simulink model "Part E"  (R2022b)
settings: Solver=VariableStepAuto  StartTime=0.0  StopTime=10.0  RelTol=1e-3
libraries: commanapbnd3 x4
settings Model: Creator=DELL  LastModifiedBy=DELL

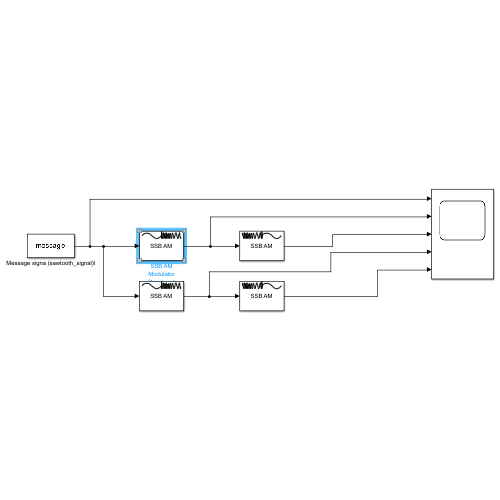
[thumbnail: Simulink's stored preview of the top-level diagram]
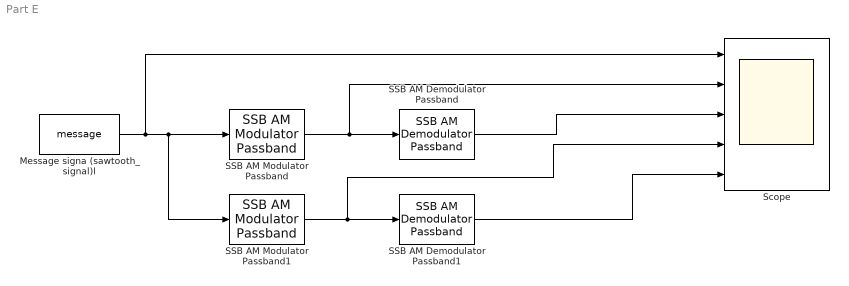
== system Part E ==
  Message signa (sawtooth_signal)l : FromWorkspace  VariableName=message  SampleTime=1/10000
  SSB AM Demodulator Passband : commanapbnd3/SSB AM Demodulator Passband  Fc=10  Ph=0  method=Butterworth  n=4  cf=300  Rp=0.1  Rs=50
  SSB AM Demodulator Passband1 : commanapbnd3/SSB AM Demodulator Passband  Fc=10  Ph=0  method=Butterworth  n=4  cf=300  Rp=0.1  Rs=50
  SSB AM Modulator Passband : commanapbnd3/SSB AM Modulator Passband  Fc=10  Ph=0  Sd=Upper  Ho=100
  SSB AM Modulator Passband1 : commanapbnd3/SSB AM Modulator Passband  Fc=10  Ph=0  Sd=Lower  Ho=100
  Scope : Scope  NumInputPorts=5
  wires:
  SSB AM Demodulator Passband/1 -> Scope/3
  SSB AM Modulator Passband/1 -> Scope/2, SSB AM Demodulator Passband/1
  Message signa (sawtooth_signal)l/1 -> Scope/1, SSB AM Modulator Passband1/1, SSB AM Modulator Passband/1
  SSB AM Demodulator Passband1/1 -> Scope/5
  SSB AM Modulator Passband1/1 -> Scope/4, SSB AM Demodulator Passband1/1
